simulink model "RLC_simulink"  (R2024a)
settings: Solver=VariableStepAuto  StartTime=0.0  StopTime=0.001  MaxStep=0.000001  RelTol=1e-3
settings Model: Creator=JUAN CARLOS  LastModifiedBy=52331

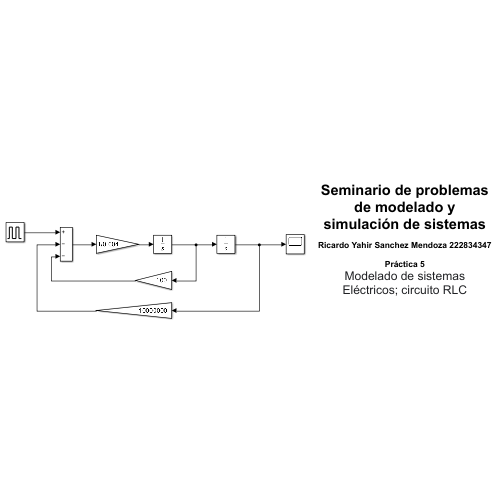
[thumbnail: Simulink's stored preview of the top-level diagram]
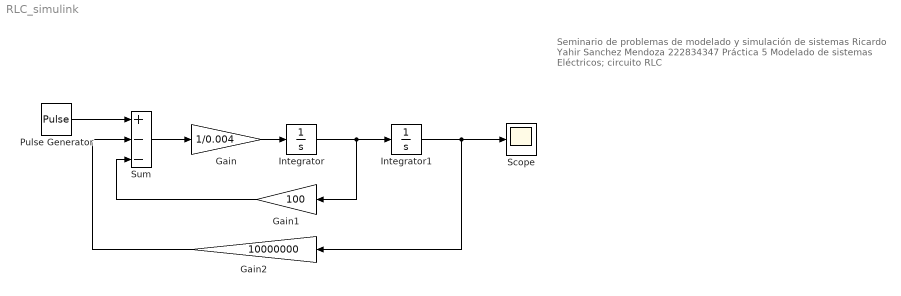
== system RLC_simulink ==
  note: Seminario de problemas de modelado y simulación de sistemas
      |
      | Ricardo Yahir Sanchez Mendoza 222834347
      |
      | Práctica 5
      | Modelado de sistemas Eléctricos; circuito RLC
  Gain : Gain  Gain=1/0.004
  Gain1 : Gain  Gain=100
  Gain2 : Gain  Gain=10000000
  Integrator : Integrator
  Integrator1 : Integrator
  Pulse Generator : DiscretePulseGenerator  PulseType=Time based  Amplitude=9  Period=0.0022  PulseWidth=50
  Scope : Scope
  Sum : Sum  Inputs=+--
  wires:
  Gain/1 -> Integrator/1
  Integrator/1 -> Gain1/1, Integrator1/1
  Integrator1/1 -> Gain2/1, Scope/1
  Pulse Generator/1 -> Sum/1
  Sum/1 -> Gain/1
  Gain1/1 -> Sum/3
  Gain2/1 -> Sum/2
